simulink model "threePhase_grid_delay"  (R2024b)
settings: Solver=VariableStepAuto  StartTime=0.0  StopTime=0.5  RelTol=1e-3
InitFcn:
  | % call the initialization file
  | predCurrCtrl_ini;
undefined symbols (not defined in the file or in its folder): Par
libraries: spsControlledVoltageSourceLib x3, spsSeriesRLCBranchLib x3, spsDCVoltageSourceLib x2, spsGroundLib x1, spsThreeLevelBridgeLib x1, spsThreePhaseVIMeasurementLib x1, sps_lib x1
settings Model: Creator=PetrosK  LastModifiedBy=horak
settings DebuggingCC: UnderspecifiedInitializationDetection=Classic  MergeDetectMultiDrivingBlocksExec=none
settings ModelReferenceCC: PropagateSignalLabelsOutOfModel=off

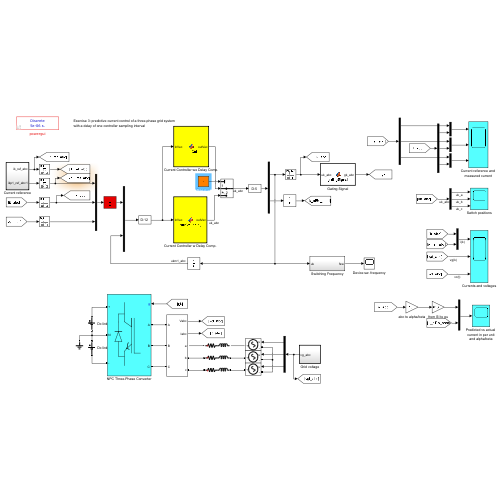
[thumbnail: Simulink's stored preview of the top-level diagram]
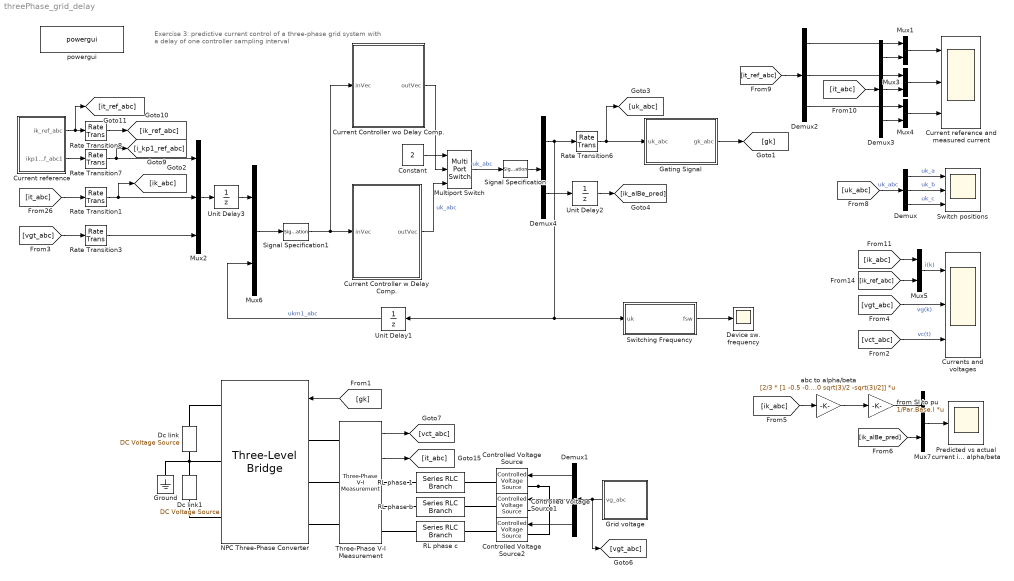
== system threePhase_grid_delay ==
  note: Exercise 3: predictive current control of a three-phase grid system
      | with a delay of one controller sampling interval
  Constant : Constant  Value=2
  Controlled Voltage Source : spsControlledVoltageSourceLib/Controlled Voltage Source  Initialize=on  Source_Type=AC  Amplitude=0  Phase=0  Frequency=0  Measurements=None
  Controlled Voltage Source1 : spsControlledVoltageSourceLib/Controlled Voltage Source  Initialize=on  Source_Type=AC  Amplitude=0  Phase=0  Frequency=0  Measurements=None
  Controlled Voltage Source2 : spsControlledVoltageSourceLib/Controlled Voltage Source  Initialize=on  Source_Type=AC  Amplitude=0  Phase=0  Frequency=0  Measurements=None
  Current Controller w Delay Comp. : MATLAB Function  TreatAsAtomicUnit=on
  Current Controller wo Delay Comp. : MATLAB Function  TreatAsAtomicUnit=on
  Current reference : Subsystem  TreatAsAtomicUnit=on
  Current reference and measured current : Scope  NumInputPorts=3
  Currents and voltages : Scope  NumInputPorts=3
  Dc link : spsDCVoltageSourceLib/DC Voltage Source  Amplitude=Par.Grid_SI.Vdc/2  Measurements=None
  Dc link1 : spsDCVoltageSourceLib/DC Voltage Source  Amplitude=Par.Grid_SI.Vdc/2  Measurements=None
  Demux{,1..3} (4 alike) : Demux  Outputs=3
  Demux4 : Demux  Outputs=[3; 2]
  Device sw. frequency : Scope
  Gating Signal : MATLAB Function  TreatAsAtomicUnit=on
  Grid voltage : Subsystem  TreatAsAtomicUnit=on
  Ground : spsGroundLib/Ground  LConnTagsString=a
  Multiport Switch : MultiPortSwitch  Inputs=2  SaturateOnIntegerOverflow=off  InputSameDT=off
  Mux{1,3..7} (6 alike) : Mux  Inputs=2
  Mux2 : Mux  Inputs=3
  NPC Three-Phase Converter : spsThreeLevelBridgeLib/Three-Level Bridge  Arms=3  SnubberResistance=1e5  SbubberCapacitance=inf  Device=IGBT / Diodes  Ron=1e-3  ForwardVoltages="[  0  0  ]"  Measurements=None
      settings: LibrarySourceBlock=sps_lib/Power Electronics/Three-Level Bridge
  Predicted vs actual current in per unit and alpha/beta : Scope
  RL phase 1 : spsSeriesRLCBranchLib/Series RLC Branch  LConnTagsString=__new0  RConnTagsString=__new0  BranchType=RL  Resistance=Par.Grid_SI.R  Inductance=Par.Grid_SI.L  SetiL0=off  InitialCurrent=0  Capacitance=1e-6  Setx0=off  InitialVoltage=0  Measurements=None
  RL phase b : spsSeriesRLCBranchLib/Series RLC Branch  LConnTagsString=__new0  RConnTagsString=__new0  BranchType=RL  Resistance=Par.Grid_SI.R  Inductance=Par.Grid_SI.L  SetiL0=off  InitialCurrent=0  Capacitance=1e-6  Setx0=off  InitialVoltage=0  Measurements=None
  RL phase c : spsSeriesRLCBranchLib/Series RLC Branch  LConnTagsString=__new0  RConnTagsString=__new0  BranchType=RL  Resistance=Par.Grid_SI.R  Inductance=Par.Grid_SI.L  SetiL0=off  InitialCurrent=0  Capacitance=1e-6  Setx0=off  InitialVoltage=0  Measurements=None
  Rate Transition{1,3,7..8} (4 alike) : RateTransition  Deterministic=off  OutPortSampleTime=Par.Ts.control
  Rate Transition6 : RateTransition  Deterministic=off  OutPortSampleTime=Par.Ts.system
  Signal Specification : SignalSpecification  Dimensions=5
  Signal Specification1 : SignalSpecification  Dimensions=12
  Switch positions : Scope  NumInputPorts=3
  Switching Frequency : Subsystem
  Three-Phase V-I Measurement : spsThreePhaseVIMeasurementLib/Three-Phase V-I Measurement  VoltageMeasurement=phase-to-ground  SetLabelV=off  LabelV=Vabc  Vpu=off  VpuLL=off  CurrentMeasurement=yes  SetLabelI=off  LabelI=Iabc  Ipu=off  Pbase=100e6  Vbase=500e3  OutputType=Complex  PhasorSimulation=off  PSBequivalent=0
  Unit Delay1 : UnitDelay  SampleTime=-1  HasFrameUpgradeWarning=on
  Unit Delay2 : UnitDelay  SampleTime=-1  HasFrameUpgradeWarning=on
  Unit Delay3 : UnitDelay  SampleTime=-1  HasFrameUpgradeWarning=on
  abc to alpha/beta : Gain  Gain=[2/3 * [1 -0.5 -0.5;0 sqrt(3)/2 -sqrt(3)/2]]  Multiplication=Matrix(K*u)  SaturateOnIntegerOverflow=on  OutDataTypeStr=Inherit: Same as input  ParamDataTypeStr=Inherit: Same as input
  from SI to pu : Gain  Gain=1/Par.Base.I  Multiplication=Matrix(K*u)  SaturateOnIntegerOverflow=on  OutDataTypeStr=Inherit: Same as input  ParamDataTypeStr=Inherit: Same as input
  powergui : sps_lib/powergui  Priority=1  SimulationMode=Discrete  SampleTime=Par.Ts.system  frequency=60  Iterations=50  frequencyindice=0  Pbase=100e6  ErrMax=1e-4  UnitsV=kV  UnitsW=MW  buscounter=0  FunctionMessages=off  echomessages=off  EnableUseOfTLC=off  CurrentSourceSwitches=off  DisableSnubberDevices=off  DisableRonSwitches=off  DisableVfSwitches=off  DisplayEquations=off  AutomaticDiscreteSolvers=off  SolverType=Tustin  Interpol=off  ExternalGateDelay=off  methode=off  Ts=0  x0status=zero  SPID=off  SwTol=0  HookPort=off  NonlinearTolerance=1e-4  nMaxIteration=100  ContinueOnMaxIteration=off  RestoreLinks=warning  ResistiveCurrentMeasurement=off  Frange=[0:2:500]  Ylog=off  Xlog=on  ShowGrid=off  save=off  variable=ZData  structure=0  ZoomFFT=off  StartTime=0.0  cycles=1  DisplayStyle=1  fundamental=60  FreqAxis=off  MaxFrequency=1000  frequencyindicesteady=1  RmsSteady=1  display=off
  wires:
  Three-Phase V-I Measurement/2 -> [it_abc]
  Demux1/1 -> Controlled Voltage Source/1
  Demux1/2 -> Controlled Voltage Source1/1
  Demux1/3 -> Controlled Voltage Source2/1
  Grid voltage/1(vg_abc) -> [vgt_abc], Demux1/1
  Three-Phase V-I Measurement/1 -> [vct_abc]
  [uk_abc] -> Demux/1  "uk_abc"
  Demux/2 -> Switch positions/2  "uk_b"
  Demux/3 -> Switch positions/3  "uk_c"
  Mux1/1 -> Current reference and measured current/1
  Mux3/1 -> Current reference and measured current/2
  Mux4/1 -> Current reference and measured current/3
  Demux2/1 -> Mux1/1
  [it_abc] -> Demux3/1
  Demux3/1 -> Mux1/2
  Demux2/2 -> Mux3/1
  Demux2/3 -> Mux4/1
  Demux3/2 -> Mux3/2
  Demux3/3 -> Mux4/2
  [it_ref_abc] -> Demux2/1
  Mux5/1 -> Currents and voltages/1  "i(k)"
  [ik_abc] -> Mux5/1
  [ik_ref_abc] -> Mux5/2
  [vgt_abc] -> Currents and voltages/2  "vg(k)"
  Demux/1 -> Switch positions/1  "uk_a"
  [gk] -> NPC Three-Phase Converter/1
  [vct_abc] -> Currents and voltages/3  "vc(t)"
  [ik_alBe_pred] -> Mux7/2
  Mux7/1 -> Predicted vs actual current in per unit and alpha/beta/1
  abc to alpha/beta/1 -> from SI to pu/1
  [ik_abc] -> abc to alpha/beta/1
  from SI to pu/1 -> Mux7/1
  Current Controller wo Delay Comp./1(outVec) -> Multiport Switch/2
  Constant/1 -> Multiport Switch/1
  Current Controller w Delay Comp./1(outVec) -> Multiport Switch/3  "uk_abc"
  Rate Transition8/1 -> [ik_ref_abc]
  Gating Signal/1(gk_abc) -> [gk]
  Mux2/1 -> Unit Delay3/1
  Current reference/2(ikp1_ref_abc1) -> Rate Transition7/1
  Unit Delay1/1 -> Mux6/2  "ukm1_abc"
  Rate Transition1/1 -> [ik_abc], Mux2/2
  Rate Transition7/1 -> Mux2/1, [i_kp1_ref_abc]
  Signal Specification/1 -> Demux4/1
  Unit Delay3/1 -> Mux6/1
  Unit Delay2/1 -> [ik_alBe_pred]
  Rate Transition3/1 -> Mux2/3
  Mux6/1 -> Signal Specification1/1
  Demux4/2 -> Unit Delay2/1
  Signal Specification1/1 -> Current Controller wo Delay Comp./1(inVec), Current Controller w Delay Comp./1(inVec)
  Rate Transition6/1 -> Gating Signal/1(uk_abc), [uk_abc]
  [it_abc] -> Rate Transition1/1
  Demux4/1 -> Unit Delay1/1, Switching Frequency/1(uk), Rate Transition6/1
  [vgt_abc] -> Rate Transition3/1
  Switching Frequency/1(fsw) -> Device sw. frequency/1
  Multiport Switch/1 -> Signal Specification/1  "uk_abc"
  Current reference/1(ik_ref_abc) -> Rate Transition8/1, [it_ref_abc]
  connections:
  NPC Three-Phase Converter/RConn2 -- Dc link1/RConn1 -- Dc link/LConn1 -- Ground/LConn1
  Controlled Voltage Source/LConn1 -- Controlled Voltage Source1/LConn1 -- Controlled Voltage Source2/LConn1
  NPC Three-Phase Converter/RConn3 -- Dc link1/LConn1
  Controlled Voltage Source1/RConn1 -- RL phase b/RConn1
  Controlled Voltage Source/RConn1 -- RL phase 1/RConn1
  Three-Phase V-I Measurement/LConn1 -- NPC Three-Phase Converter/LConn1
  NPC Three-Phase Converter/RConn1 -- Dc link/RConn1
  Controlled Voltage Source2/RConn1 -- RL phase c/RConn1
  Three-Phase V-I Measurement/LConn3 -- NPC Three-Phase Converter/LConn3
  NPC Three-Phase Converter/LConn2 -- Three-Phase V-I Measurement/LConn2
  RL phase b/LConn1 -- Three-Phase V-I Measurement/RConn2
  RL phase c/LConn1 -- Three-Phase V-I Measurement/RConn3
  RL phase 1/LConn1 -- Three-Phase V-I Measurement/RConn1

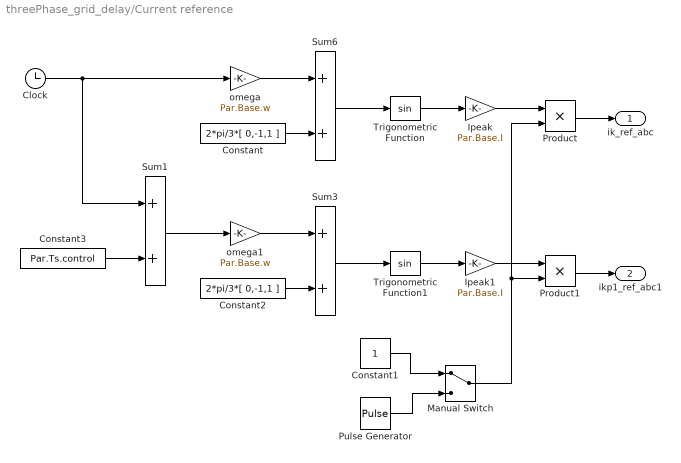
== system threePhase_grid_delay/Current reference ==
  Clock : Clock
  Constant : Constant  Value=2*pi/3*[ 0,-1,1 ]
  Constant1 : Constant
  Constant2 : Constant  Value=2*pi/3*[ 0,-1,1 ]
  Constant3 : Constant  Value=Par.Ts.control
  Ipeak : Gain  Gain=Par.Base.I  SaturateOnIntegerOverflow=on  OutDataTypeStr=Inherit: Same as input  ParamDataTypeStr=Inherit: Same as input
  Ipeak1 : Gain  Gain=Par.Base.I  SaturateOnIntegerOverflow=on  OutDataTypeStr=Inherit: Same as input  ParamDataTypeStr=Inherit: Same as input
  Manual Switch : ManualSwitch
  Product : Product
  Product1 : Product
  Pulse Generator : DiscretePulseGenerator  PulseType=Time based  Period=0.02  PulseWidth=50
  Sum1 : Sum  InputSameDT=on  SaturateOnIntegerOverflow=on  OutDataTypeStr=Inherit: Same as first input
  Sum3 : Sum  InputSameDT=on  SaturateOnIntegerOverflow=on  OutDataTypeStr=Inherit: Same as first input
  Sum6 : Sum  InputSameDT=on  SaturateOnIntegerOverflow=on  OutDataTypeStr=Inherit: Same as first input
  Trigonometric Function : Trigonometry
  Trigonometric Function1 : Trigonometry
  omega : Gain  Gain=Par.Base.w  SaturateOnIntegerOverflow=on  OutDataTypeStr=Inherit: Same as input  ParamDataTypeStr=Inherit: Same as input
  omega1 : Gain  Gain=Par.Base.w  SaturateOnIntegerOverflow=on  OutDataTypeStr=Inherit: Same as input  ParamDataTypeStr=Inherit: Same as input
  ik_ref_abc : Outport
  ikp1_ref_abc1 : Outport  Port=2
  wires:
  Sum6/1 -> Trigonometric Function/1
  Constant/1 -> Sum6/2
  omega/1 -> Sum6/1
  Trigonometric Function/1 -> Ipeak/1
  Sum3/1 -> Trigonometric Function1/1
  Constant2/1 -> Sum3/2
  omega1/1 -> Sum3/1
  Trigonometric Function1/1 -> Ipeak1/1
  Clock/1 -> Sum1/1, omega/1
  Sum1/1 -> omega1/1
  Constant3/1 -> Sum1/2
  Ipeak/1 -> Product/1
  Ipeak1/1 -> Product1/1
  Product1/1 -> ikp1_ref_abc1/1
  Product/1 -> ik_ref_abc/1
  Manual Switch/1 -> Product/2, Product1/2
  Pulse Generator/1 -> Manual Switch/2
  Constant1/1 -> Manual Switch/1

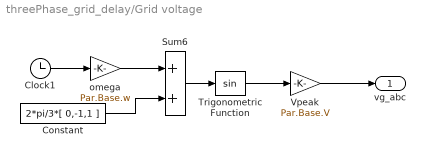
== system threePhase_grid_delay/Grid voltage ==
  Clock1 : Clock
  Constant : Constant  Value=2*pi/3*[ 0,-1,1 ]
  Sum6 : Sum  InputSameDT=on  SaturateOnIntegerOverflow=on  OutDataTypeStr=Inherit: Same as first input
  Trigonometric Function : Trigonometry
  Vpeak : Gain  Gain=Par.Base.V  SaturateOnIntegerOverflow=on  OutDataTypeStr=Inherit: Same as input  ParamDataTypeStr=Inherit: Same as input
  omega : Gain  Gain=Par.Base.w  SaturateOnIntegerOverflow=on  OutDataTypeStr=Inherit: Same as input  ParamDataTypeStr=Inherit: Same as input
  vg_abc : Outport
  wires:
  Sum6/1 -> Trigonometric Function/1
  Constant/1 -> Sum6/2
  Clock1/1 -> omega/1
  omega/1 -> Sum6/1
  Trigonometric Function/1 -> Vpeak/1
  Vpeak/1 -> vg_abc/1

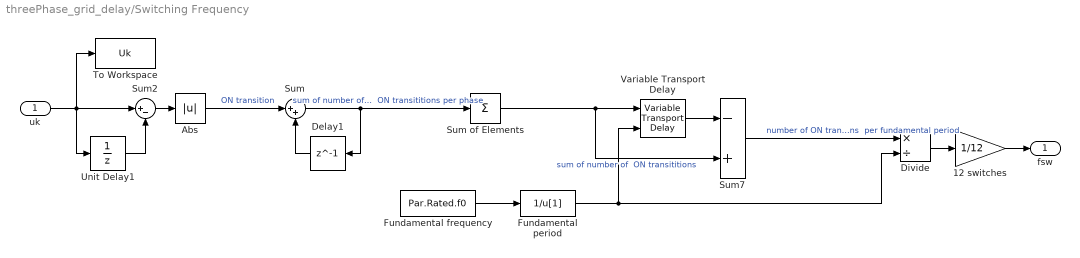
== system threePhase_grid_delay/Switching Frequency ==
  uk : Inport
  12 switches : Gain  Gain=1/12
  Abs : Abs  SaturateOnIntegerOverflow=off
  Delay1 : Delay  DelayLength=1  InitialCondition=0
  Divide : Product  Inputs=*/
  Fundamental frequency : Constant  Value=Par.Rated.f0
  Fundamental period : Fcn  Expr=1/u[1]
  Sum : Sum  Inputs=|++
  Sum of Elements : Sum  Inputs=+
  Sum2 : Sum  Inputs=|+-
  Sum7 : Sum  Inputs=-+  InputSameDT=on  SaturateOnIntegerOverflow=on  OutDataTypeStr=Inherit: Same as first input
  To Workspace : ToWorkspace  VariableName=Uk  SaveFormat=Structure With Time  SampleTime=-1
  Unit Delay1 : UnitDelay  SampleTime=-1  HasFrameUpgradeWarning=on
  Variable Transport Delay : VariableTransportDelay  VariableDelayType=Variable transport delay  MaximumDelay=0.05  MaximumPoints=2048*4  PadeOrder=2
  fsw : Outport
  wires:
  Sum/1 -> Sum of Elements/1, Delay1/1  "sum of number of  ON transititions per phase"
  Variable Transport Delay/1 -> Sum7/1
  Delay1/1 -> Sum/2
  Fundamental frequency/1 -> Fundamental period/1
  Fundamental period/1 -> Divide/2, Variable Transport Delay/2
  Sum7/1 -> Divide/1  "number of ON transitions  per fundamental period"
  uk/1 -> To Workspace/1, Sum2/1, Unit Delay1/1
  Unit Delay1/1 -> Sum2/2
  Sum2/1 -> Abs/1
  Abs/1 -> Sum/1  "ON transition"
  Divide/1 -> 12 switches/1
  12 switches/1 -> fsw/1
  Sum of Elements/1 -> Variable Transport Delay/1, Sum7/2  "sum of number of  ON transititions"

== matlab function threePhase_grid_delay/Gating Signal ==
  data: uk_abc input; gk_abc output
function gk_abc = gatingSignal(uk_abc)

% Translate the three-phase switch position u_abc(k) = {-1, 0, 1}^3 into 
% a gating signal for the three-level three-phase leg g_abc(k)
%
% Model Predictive Control of Power Electronic Systems, TAU, Tampere
% Petros Karamanakos, September 2025

gk_abc = [gatingSignal_1ph(uk_abc(1));
          gatingSignal_1ph(uk_abc(2));
          gatingSignal_1ph(uk_abc(3))];

return


function gk = gatingSignal_1ph(uk)

% single-phase gating signal according to Table 2.3
if uk == 1
    gk = [1 1 0 0]';
elseif uk == 0
    gk = [0 1 1 0]';
elseif uk == -1
    gk = [0 0 1 1]';
else
    error('unknown switch position');
end

== matlab function threePhase_grid_delay/Current Controller w Delay Comp. ==
  data: inVec input; outVec output; Par parameter
function outVec = currCtrl_delay(inVec, Par)

% Predictive current controller for a three-phase grid system with a 
% prediction horizon of one step with delay compensation
%
% Model Predictive Control of Power Electronic Systems, TAU, Tampere
% Petros Karamanakos, September 2025
% 
% global Par

% interface
ik_ref_abc = inVec(1:3);	% three-phase current reference at time step k
ikm1_abc = inVec(4:6);    	% three-phase current measurement at time step k-1
vgkm1_abc = inVec(7:9);    	% three-phase grid voltage measurement at time step k-1
ukm1_abc = inVec(10:12);   	% previous three-phase switch position applied at time step k-1

% turn the inputs into the per unit system and the stationary orthogonal 
% reference frame
ab_ik_ref = Par.K* ik_ref_abc/Par.Base.I; 
ab_ikm1 =Par.K*ikm1_abc/Par.Base.I  ;       
ab_vgkm1 =Par.K* vgkm1_abc/Par.Base.V;    

% implement the predictive current controller
% **** to be added ****
sm=sum(abs(ukm1_abc))+1;% 0 1 2 3 +1
pole_pocet=[3*3*3, 3*3*2, 3*2*2, 2*2*2];
n=pole_pocet(sm);

iter=1;
pos_u=zeros(n,3);

for i=-1:1
    for j=-1:1
        for k=-1:1
            tmp=[i,j,k];
            if(max(abs(tmp-ukm1_abc'))<2)
                pos_u(iter,:)=tmp;
                iter=iter+1;
            end
            
        end
    end
end
ik_pred=Par.Ctr.A*ab_ikm1+Par.Ctr.B1*ukm1_abc+Par.Ctr.B2*ab_vgkm1;

J=ones(size(pos_u,1),1);
ik1_pred=zeros(2,n);
for i=1:n
    ik1_pred(:,i)=Par.Ctr.A*ik_pred+Par.Ctr.B1*pos_u(i,:)'+Par.Ctr.B2*ab_vgkm1;

    J(i)=norm(ik1_pred(:,i)-ab_ik_ref,2)^2+Par.Ctr.lambdaU *norm(ukm1_abc-pos_u(i,:)',1);
end
[~,index]=min(J);

uk_abc=pos_u(index,:);

% for the chosen switch position: 
% compute the predicted current in pu and alpha/beta at the next time step
% ikp1 = ik1_pred(:,index)  % **** to be added ****
ikp1= ik1_pred(:,index);

% output interface
outVec = [uk_abc'; ikp1];

return

== matlab function threePhase_grid_delay/Current Controller wo Delay Comp. ==
  data: inVec input; outVec output; Par parameter
function outVec = currCtrl(inVec, Par)

% Predictive current controller for a three-phase grid system with a 
% prediction horizon of one step
%
% Model Predictive Control of Power Electronic Systems, TAU, Tampere
% Petros Karamanakos, September 2025

% interface
ikp1_ref_abc = inVec(1:3);	% three-phase current reference at time step k+1
ik_abc = inVec(4:6);        % three-phase current measurement at time step k
vgk_abc = inVec(7:9);    	% three-phase grid voltage measurement at time step k
ukm1_abc = inVec(10:12);   	% previous three-phase switch position applied at time step k-1

% turn the inputs into the per unit system and the stationary orthogonal 
% reference frame
ab_ikp1_ref = Par.K* ikp1_ref_abc/Par.Base.I; 	% three-phase current reference at time step k+1
ab_ik =Par.K*ik_abc/Par.Base.I  ;        % three-phase current measurement at time step k
ab_vgk =Par.K* vgk_abc/Par.Base.V;    	% three-phase grid voltage measurement at time step k


% implement the predictive current controller
% **** to be added ****
sm=sum(abs(ukm1_abc))+1;% 0 1 2 3 +1
pole_pocet=[3*3*3, 3*3*2, 3*2*2, 2*2*2];
n=pole_pocet(sm);

iter=1;
pos_u=zeros(n,3);

for i=-1:1
    for j=-1:1
        for k=-1:1
            tmp=[i,j,k];
            if(max(abs(tmp-ukm1_abc'))<2)
                pos_u(iter,:)=tmp;
                iter=iter+1;
            end
            
        end
    end
end

J=ones(size(pos_u,1),1);
ik1_pred=zeros(2,n);
for i=1:n
    ik1_pred(:,i)=Par.Ctr.A*ab_ik+Par.Ctr.B1*pos_u(i,:)'+Par.Ctr.B2*ab_vgk;
    J(i)=norm(ik1_pred(:,i)-ab_ikp1_ref,2)^2+Par.Ctr.lambdaU *norm(ukm1_abc-pos_u(i,:)',1);
end
[~,index]=min(J);

uk_abc=pos_u(index,:);

% for the chosen switch position: 
% compute the predicted current in pu and alpha/beta at the next time step
% ikp1 = ik1_pred(:,index)  % **** to be added ****
ikp1= ik1_pred(:,index);

% output interface
outVec = [uk_abc'; ikp1];
return
